simulink model "lab10q1"  (Simulink 7.1)
settings: Solver=ode45  StartTime=0.0  StopTime=10  RelTol=1e-3
InitFcn:
  | A = [1 1 0;-12 0 1;20 0 0];
  | 
  | B1 = [0;1;1];
  | 
  | C = [21 -1 1;1 0 0 ;0 1 0;0 0 1];
  | 
  | D=[0; 0; 0; 0];
settings Model: Creator=ALUNO  LastModifiedBy=ALUNO

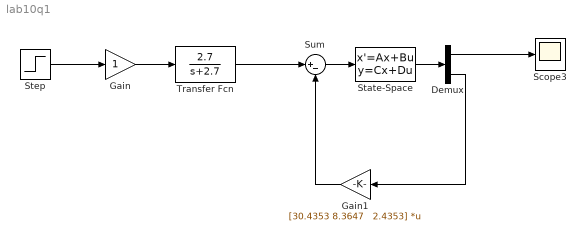
== system lab10q1 ==
  Demux : Demux  Outputs=[1 3]
  Gain : Gain  ParameterDataType=sfix(16)  ParameterScaling=2^0  OutDataType=sfix(16)  OutScaling=2^0
  Gain1 : Gain  Orientation=left  Gain="[30.4353 8.3647   2.4353]"  Multiplication=Matrix(K*u) (u vector)  ParameterDataType=sfix(16)  ParameterScaling=2^0  OutDataType=sfix(16)  OutScaling=2^0
  Scope3 : Scope
      settings: TimeRange=100  YMin=0  YMax=1.2e+068  SaveName=ScopeData3
  State-Space : StateSpace  A=A  B=B1  C=C  D=D
  Step : Step  Time=0  SampleTime=0
  Sum : Sum  Inputs=|+-  OutDataType=sfix(16)  OutScaling=2^0
  Transfer Fcn : TransferFcn  InitFcn=|  Numerator=[2.7]  Denominator=[1 2.7]
      | J=0.5;
      | B=0;  
      | O=10; 
      | r=1;  
      | R=49; 
      | K=4;  
      | E=9;
  wires:
  State-Space/1 -> Demux/1
  Sum/1 -> State-Space/1
  Gain1/1 -> Sum/2
  Demux/2 -> Gain1/1
  Step/1 -> Gain/1
  Gain/1 -> Transfer Fcn/1
  Transfer Fcn/1 -> Sum/1
  Demux/1 -> Scope3/1
